simulink model "nonlinear_model"  (R2016b)
settings: Solver=VariableStepAuto  StartTime=0.0  StopTime=4  RelTol=1e-3
undefined symbols (not defined in the file): j_e, j_lambda, j_p, k_pd, k_pp, k_rp, L1, L2, L3, L4
settings Model: Creator=Kevin K. Kaldvansvik  LastModifiedBy=Kevin K. Kaldvansvik

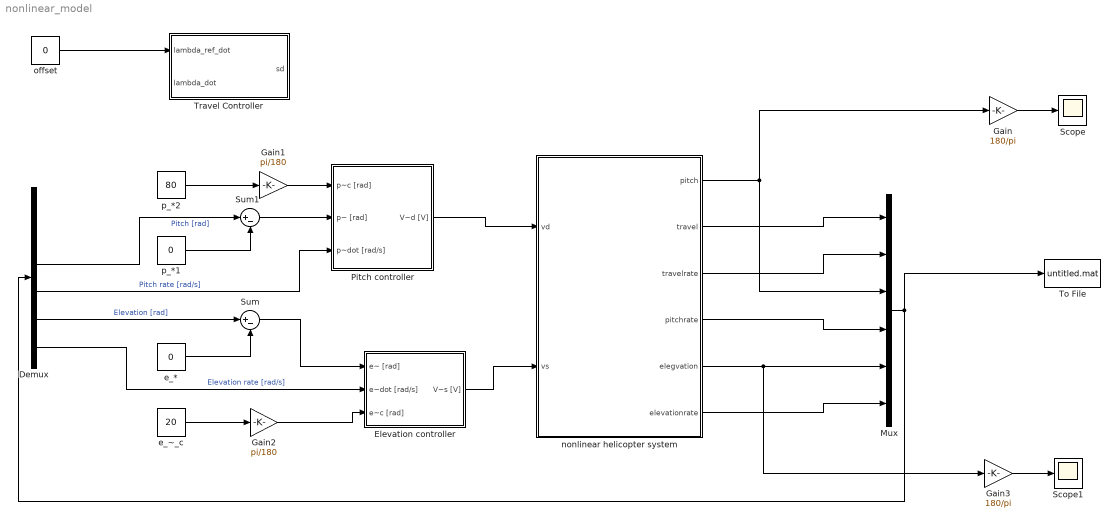
== system nonlinear_model ==
  Demux : Demux  Outputs=6
  Elevation controller : Subsystem
  Gain : Gain  Gain=180/pi
  Gain1 : Gain  Gain=pi/180
  Gain2 : Gain  Gain=pi/180
  Gain3 : Gain  Gain=180/pi
  Mux : Mux  Inputs=6
  Pitch controller : Subsystem
  Scope : Scope
  Scope1 : Scope
  Sum : Sum  Inputs=|+-
  Sum1 : Sum  Inputs=|+-
  To File : ToFile  MatrixName=kp_v1
  Travel Controller : Subsystem
  e_* : Constant  Value=0
  e_~_c : Constant  Value=20
  nonlinear helicopter system : Subsystem
  offset : Constant  Value=0
  p_*1 : Constant  Value=0
  p_*2 : Constant  Value=80
  wires:
  e_~_c/1 -> Gain2/1
  e_*/1 -> Sum/2
  Demux/6 -> Elevation controller/2(e~dot [rad/s])  "Elevation rate [rad/s]"
  Sum/1 -> Elevation controller/1(e~ [rad])
  p_*1/1 -> Sum1/2
  Sum1/1 -> Pitch controller/2(p~ [rad])
  Demux/4 -> Pitch controller/3(p~dot [rad/s])  "Pitch rate [rad/s]"
  Mux/1 -> To File/1, Demux/1
  Demux/5 -> Sum/1  "Elevation [rad]"
  Demux/3 -> Sum1/1  "Pitch [rad]"
  offset/1 -> Travel Controller/1("lambda_ref_dot ")
  Gain/1 -> Scope/1
  p_*2/1 -> Gain1/1
  Gain1/1 -> Pitch controller/1(p~c [rad])
  Gain2/1 -> Elevation controller/3(e~c [rad])
  Gain3/1 -> Scope1/1
  nonlinear helicopter system/5(elegvation) -> Mux/5, Gain3/1
  nonlinear helicopter system/1(pitch) -> Mux/3, Gain/1
  Pitch controller/1(V~d [V]) -> nonlinear helicopter system/1(vd)
  Elevation controller/1(V~s [V]) -> nonlinear helicopter system/2(vs)
  nonlinear helicopter system/2(travel) -> Mux/1
  nonlinear helicopter system/3(travelrate) -> Mux/2
  nonlinear helicopter system/4(pitchrate) -> Mux/4
  nonlinear helicopter system/6(elevationrate) -> Mux/6

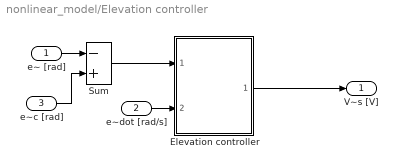
== system nonlinear_model/Elevation controller ==
  e~ [rad] : Inport
  e~dot [rad/s] : Inport  Port=2
  e~c [rad] : Inport  Port=3
  Elevation controller : Subsystem
  Sum : Sum  Inputs=-+  SaturateOnIntegerOverflow=on  InputSameDT=on  OutDataTypeStr=Inherit: Same as first input
  V~s [V] : Outport  InitialOutput=0
  wires:
  Sum/1 -> Elevation controller/1(e~ [rad])
  Elevation controller/1(V~_s [V]) -> V~s [V]/1
  e~ [rad]/1 -> Sum/1
  e~dot [rad/s]/1 -> Elevation controller/2(e~_dot [rad/s])
  e~c [rad]/1 -> Sum/2

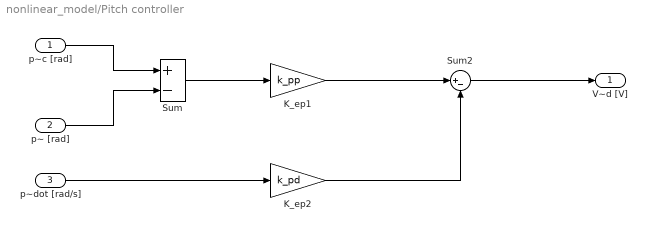
== system nonlinear_model/Pitch controller ==
  p~c [rad] : Inport
  p~ [rad] : Inport  Port=2
  p~dot [rad/s] : Inport  Port=3
  K_ep1 : Gain  Gain=k_pp  SaturateOnIntegerOverflow=on  OutDataTypeStr=Inherit: Same as input  ParamDataTypeStr=Inherit: Same as input
  K_ep2 : Gain  Gain=k_pd  SaturateOnIntegerOverflow=on  OutDataTypeStr=Inherit: Same as input  ParamDataTypeStr=Inherit: Same as input
  Sum : Sum  Inputs=+-  SaturateOnIntegerOverflow=on  InputSameDT=on  OutDataTypeStr=Inherit: Same as first input
  Sum2 : Sum  Inputs=|+-
  V~d [V] : Outport  InitialOutput=0
  wires:
  p~c [rad]/1 -> Sum/1
  p~ [rad]/1 -> Sum/2
  Sum/1 -> K_ep1/1
  p~dot [rad/s]/1 -> K_ep2/1
  K_ep1/1 -> Sum2/1
  K_ep2/1 -> Sum2/2
  Sum2/1 -> V~d [V]/1

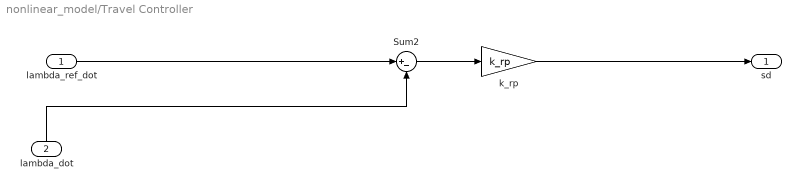
== system nonlinear_model/Travel Controller ==
  "lambda_ref_dot " : Inport
  "lambda_dot " : Inport  Port=2
  Sum2 : Sum  Inputs=|+-
  k_rp : Gain  Gain=k_rp
  "sd " : Outport
  wires:
  k_rp/1 -> "sd "/1
  Sum2/1 -> k_rp/1
  "lambda_ref_dot "/1 -> Sum2/1
  "lambda_dot "/1 -> Sum2/2

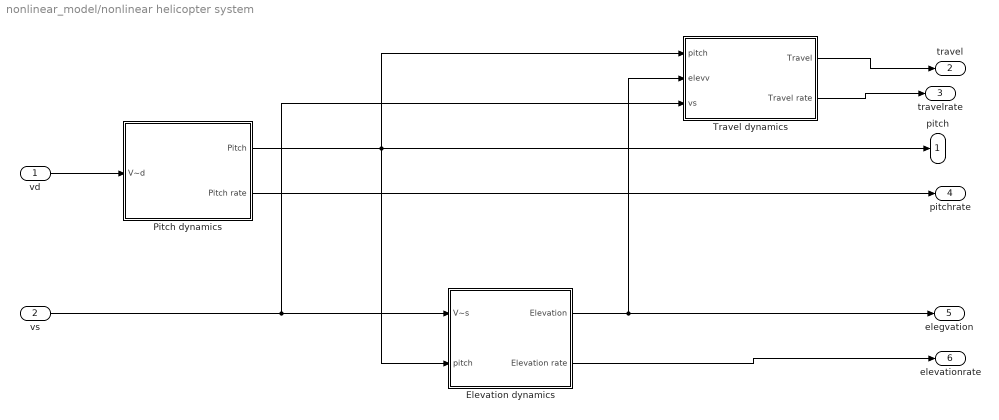
== system nonlinear_model/nonlinear helicopter system ==
  vd : Inport
  vs : Inport  Port=2
  Elevation dynamics : Subsystem
  Pitch dynamics : Subsystem
  Travel dynamics : Subsystem
  pitch : Outport
  travel : Outport  Port=2
  travelrate : Outport  Port=3
  pitchrate : Outport  Port=4
  elegvation : Outport  Port=5
  elevationrate : Outport  Port=6
  wires:
  vd/1 -> Pitch dynamics/1(V~d)
  Elevation dynamics/1(Elevation) -> Travel dynamics/2(elevv), elegvation/1
  Pitch dynamics/2(Pitch rate) -> pitchrate/1
  vs/1 -> Elevation dynamics/1(V~s), Travel dynamics/3(vs)
  Pitch dynamics/1(Pitch) -> Elevation dynamics/2(pitch), Travel dynamics/1(pitch), pitch/1
  Travel dynamics/2(Travel rate) -> travelrate/1
  Travel dynamics/1(Travel) -> travel/1
  Elevation dynamics/2(Elevation rate) -> elevationrate/1

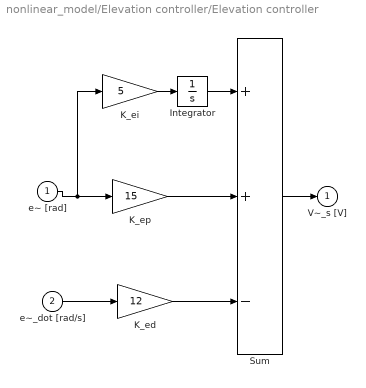
== system nonlinear_model/Elevation controller/Elevation controller ==
  e~ [rad] : Inport
  e~_dot [rad/s] : Inport  Port=2
  Integrator : Integrator  LimitOutput=on
  K_ed : Gain  Gain=12  SaturateOnIntegerOverflow=on  OutDataTypeStr=Inherit: Same as input  ParamDataTypeStr=Inherit: Same as input
  K_ei : Gain  Gain=5  SaturateOnIntegerOverflow=on  OutDataTypeStr=Inherit: Same as input  ParamDataTypeStr=Inherit: Same as input
  K_ep : Gain  Gain=15  SaturateOnIntegerOverflow=on  OutDataTypeStr=Inherit: Same as input  ParamDataTypeStr=Inherit: Same as input
  Sum : Sum  Inputs=++-  SaturateOnIntegerOverflow=on  InputSameDT=on  OutDataTypeStr=Inherit: Same as first input
  V~_s [V] : Outport  InitialOutput=0
  wires:
  K_ei/1 -> Integrator/1
  Integrator/1 -> Sum/1
  Sum/1 -> V~_s [V]/1
  e~_dot [rad/s]/1 -> K_ed/1
  K_ed/1 -> Sum/3
  K_ep/1 -> Sum/2
  e~ [rad]/1 -> K_ep/1, K_ei/1

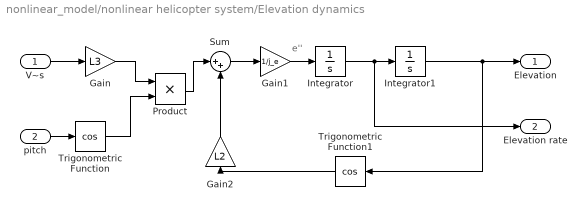
== system nonlinear_model/nonlinear helicopter system/Elevation dynamics ==
  note: e''
  V~s : Inport
  pitch : Inport  Port=2
  Gain : Gain  Gain=L3
  Gain1 : Gain  Gain=1/j_e
  Gain2 : Gain  Gain=L2
  Integrator : Integrator
  Integrator1 : Integrator
  Product : Product
  Sum : Sum  Inputs=|++
  Trigonometric Function : Trigonometry  Operator=cos
  Trigonometric Function1 : Trigonometry  Operator=cos
  Elevation : Outport
  Elevation rate : Outport  Port=2
  wires:
  Integrator/1 -> Elevation rate/1, Integrator1/1
  V~s/1 -> Gain/1
  Integrator1/1 -> Trigonometric Function1/1, Elevation/1
  Gain/1 -> Product/1
  Sum/1 -> Gain1/1
  Gain1/1 -> Integrator/1
  Product/1 -> Sum/1
  pitch/1 -> Trigonometric Function/1
  Trigonometric Function/1 -> Product/2
  Trigonometric Function1/1 -> Gain2/1
  Gain2/1 -> Sum/2

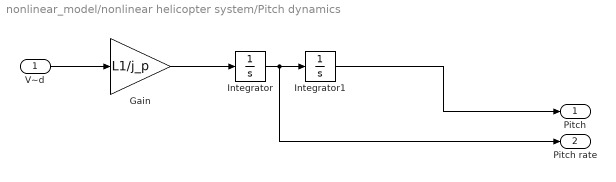
== system nonlinear_model/nonlinear helicopter system/Pitch dynamics ==
  V~d : Inport
  Gain : Gain  Gain=L1/j_p
  Integrator : Integrator
  Integrator1 : Integrator
  Pitch : Outport
  Pitch rate : Outport  Port=2
  wires:
  Integrator/1 -> Pitch rate/1, Integrator1/1
  Integrator1/1 -> Pitch/1
  V~d/1 -> Gain/1
  Gain/1 -> Integrator/1

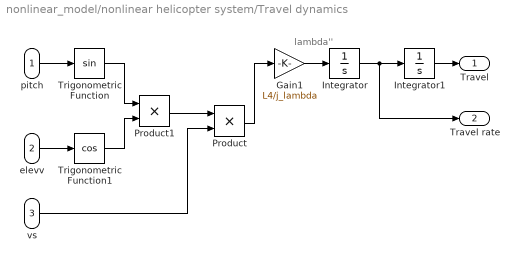
== system nonlinear_model/nonlinear helicopter system/Travel dynamics ==
  note: lambda''
  pitch : Inport
  elevv : Inport  Port=2
  vs : Inport  Port=3
  Gain1 : Gain  Gain=L4/j_lambda
  Integrator : Integrator
  Integrator1 : Integrator
  Product : Product
  Product1 : Product
  Trigonometric Function : Trigonometry
  Trigonometric Function1 : Trigonometry  Operator=cos
  Travel : Outport
  Travel rate : Outport  Port=2
  wires:
  Integrator1/1 -> Travel/1
  Integrator/1 -> Integrator1/1, Travel rate/1
  pitch/1 -> Trigonometric Function/1
  Gain1/1 -> Integrator/1
  elevv/1 -> Trigonometric Function1/1
  Product/1 -> Gain1/1
  Trigonometric Function/1 -> Product1/1
  Trigonometric Function1/1 -> Product1/2
  vs/1 -> Product/2
  Product1/1 -> Product/1
